simulink model "pid1DOF"  (R2018a)
settings: Solver=FixedStepAuto  StartTime=0.0  StopTime=150  FixedStep=.1  RelTol=1e-3
libraries: robotlib x3, vrlib x1, simulink x1
settings Model: SimulationMode=accelerator  EnablePacing=on  PacingRate=3  Creator=thedoctor  LastModifiedBy=transmogrifier

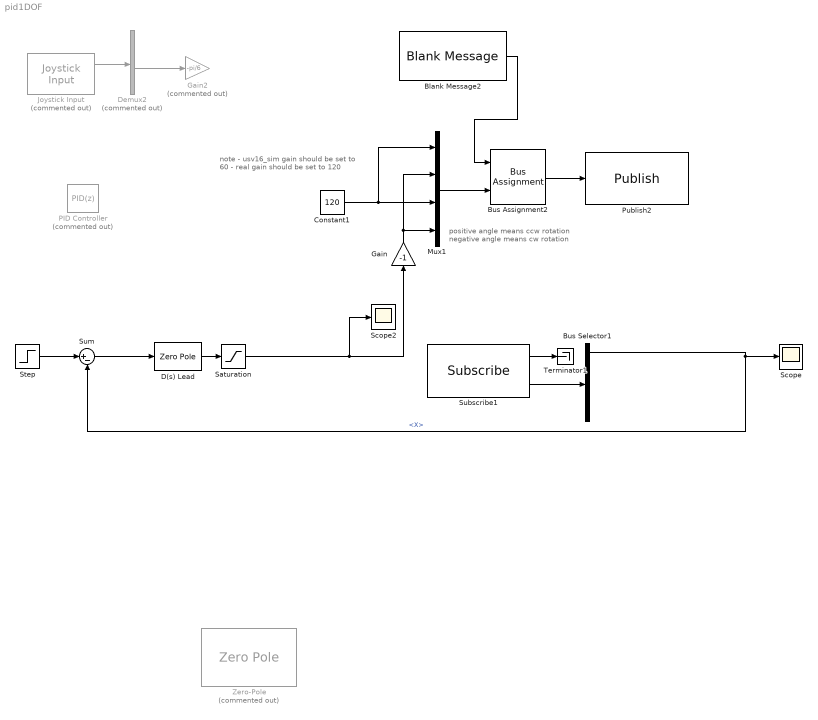
== system pid1DOF ==
  note: note
      |  - usv16_sim gain should be set to 60
      |  - real gain should be set to 120
  note: positive angle means ccw rotation
      | negative angle means cw rotation
  Blank Message2 : robotlib/Blank Message  SourceLibraryInfo=This block requires Robotics System Toolbox  messageType=usv16_msgs/Usv16ActuatorInputs  SampleTime=0.1
      settings: SourceProductBaseCode=RO
  Bus Assignment2 : BusAssignment  AssignedSignals=ActuatorInputs
  Bus Selector1 : BusSelector  OutputSignals=Pose.X,Pose.Y,Vel.Linear.X,Vel.Linear.Y
  Constant1 : Constant  Value=120
  D(s) Lead : ZeroPole  Zeros=[-.26]  Poles=[-22]  Gain=[45]
  Demux2 : Demux  Commented=on  Outputs=6
  Gain : Gain  Gain=-1
  Gain2 : Gain  Commented=on  Gain=-pi/6
  Joystick Input : vrlib/Joystick Input  Commented=on  joyid=1  adjustports=on  forcefeed=off
      settings: SourceProductBaseCode=VR
  Mux1 : Mux
  PID Controller : simulink/Continuous/PID Controller  Commented=on  Controller=PID  TimeDomain=Discrete-time  SampleTime=.1  IntegratorMethod=Backward Euler  FilterMethod=Backward Euler  Form=Parallel  UseFilter=on  ControllerParametersSource=internal  P=1.1  I=.005  D=2  N=73.2854976407746  InitialConditionSource=internal  InitialConditionForIntegrator=0  InitialConditionForFilter=0  ExternalReset=none  LimitOutput=off  UpperSaturationLimit=inf  LowerSaturationLimit=-inf  LinearizeAsGain=on  AntiWindupMode=none  Kb=1  TrackingMode=off  Kt=1  PParamMin=[]  PParamMax=[]  IParamMin=[]  IParamMax=[]  DParamMin=[]  DParamMax=[]  NParamMin=[]  NParamMax=[]  KbParamMin=[]  KbParamMax=[]  KtParamMin=[]  KtParamMax=[]  POutMin=[]  POutMax=[]  IOutMin=[]  IOutMax=[]  DOutMin=[]  DOutMax=[]  NOutMin=[]  NOutMax=[]  KbOutMin=[]  KbOutMax=[]  KtOutMin=[]  KtOutMax=[]  IntegratorOutMin=[]  IntegratorOutMax=[]  FilterOutMin=[]  FilterOutMax=[]  SumOutMin=[]  SumOutMax=[]  SumI1OutMin=[]  SumI1OutMax=[]  SumI2OutMin=[]  SumI2OutMax=[]  SumI3OutMin=[]  SumI3OutMax=[]  SumDOutMin=[]  SumDOutMax=[]  SaturationOutMin=[]  SaturationOutMax=[]  IntegratorContinuousStateAttributes=''  IntegratorStateMustResolveToSignalObject=off  IntegratorRTWStateStorageClass=Auto  FilterContinuousStateAttributes=''  FilterStateMustResolveToSignalObject=off  FilterRTWStateStorageClass=Auto  DifferentiatorICPrevScaledInput=0  DifferentiatorOutMin=[]  DifferentiatorOutMax=[]  FilterDiffOutCoefMin=[]  FilterDiffOutCoefMax=[]  SumDenOutMin=[]  SumDenOutMax=[]  SumNumOutMin=[]  SumNumOutMax=[]  ReciprocalOutMin=[]  ReciprocalOutMax=[]  DivideOutMin=[]  DivideOutMax=[]  TunerSelectOption=Transfer Function Based (PID Tuner App)
  Publish2 : robotlib/Publish  SourceLibraryInfo=This block requires Robotics System Toolbox  topicSource=Select from ROS network  topic=/ship/actuation  messageType=usv16_msgs/Usv16ActuatorInputs  messageQueueLength=1
      settings: SourceProductBaseCode=RO
  Saturation : Saturate  UpperLimit=pi/12  LowerLimit=-pi/12
  Scope : Scope
  Scope2 : Scope
  Step : Step  Time=30  After=4  SampleTime=0
  Subscribe1 : robotlib/Subscribe  SourceLibraryInfo=This block requires Robotics System Toolbox  topicSource=Select from ROS network  topic=/ship/state  messageType=usv16_msgs/Usv16State  sampleTime=0.1  messageQueueLength=1
      settings: SourceProductBaseCode=RO
  Sum : Sum  Inputs=|+-
  Terminator1 : Terminator
  Zero-Pole : ZeroPole  Commented=on  Zeros=[]  Poles=[0 0 -10/4]  Gain=1.5/9
  wires:
  D(s) Lead/1 -> Saturation/1
  Sum/1 -> D(s) Lead/1
  Bus Selector1/1 -> Sum/2, Scope/1  "<X>"
  Step/1 -> Sum/1
  Constant1/1 -> Mux1/1, Mux1/3
  Gain/1 -> Mux1/4, Mux1/2
  Bus Assignment2/1 -> Publish2/1
  Blank Message2/1 -> Bus Assignment2/1
  Mux1/1 -> Bus Assignment2/2
  Demux2/4 -> Gain2/1
  Joystick Input/1 -> Demux2/1
  Subscribe1/1 -> Terminator1/1
  Subscribe1/2 -> Bus Selector1/1
  Saturation/1 -> Gain/1, Scope2/1
